simulink model "Filter_attivo"  (R2016b)
settings: Solver=ode23t  StartTime=0.0  StopTime=2.4  MaxStep=1e-4  RelTol=1e-3  EnableMultiTasking=on
values from neighbouring files (symbols this model uses):
  ampiezza_rete = 150/sqrt(3)    [Data.m]    (also in taratura.m)
  C = 2.2e-3    (= 0.0022)    [Data.m]
  C_raddr = 600e-6    (= 0.0006)    [Data.m]
  f = 50    [Data.m]    (also in Spettro_complesso.m = bar(-fp((26:25:25000-25)),PyTHD(length(PyTHD)-1:-1:length(Py)
  f_am = 500    [Data.m]
  h = Lagrange_coef(f,1/Tc)    [Data.m]    (also in Lagrange_coef.m = NaN(4,round(fc/f1*0.5)))
  h_rit = Lagrange_coef_rit(1.5)    [Data.m]
  k_interno = 0.99    [tuning.m]
  k_par_AM = 10    [Data.m]
  ki_PI = 0.2    [Data.m]
  ki_PLL = 1000    [Data.m]
  ki_ris = 47.5*2    (= 95)    [Data.m]
  kp_PI = 1.57    [Data.m]
  kp_PLL = 0.9    [Data.m]
  kp_ris = 47.5*0.089*2    (= 8.455)    [Data.m]
  L_disaccoppiamento = 2*1.18e-3    (= 0.00236)    [Data.m]    (also in taratura.m)
  L_rete = 4e-3    (= 0.004)    [Data.m]    (also in tuning.m)
  max_PI = 8    [Data.m]
  max_PLL = 1000    [Data.m]
  min_PI = -8    [Data.m]
  min_PLL = -1000    [Data.m]
  Notch_z = 1-Peaking_z    [Data.m]
  Notch_z_AM1 = 1-Peaking_z_AM1    [Notch.m]
  peak_rete = Peaking(f,1/Tc,0.1)    [Data.m]
  Peaking_dir1_d = c2d(Peaking_dir1_s,1/fs,'tustin')    [semipeaking.m]
  pendenza = 1000    [Data.m]
  R_carico = 50    [Data.m]
  R_disaccoppiamento = 2*13e-3    (= 0.026)    [Data.m]    (also in taratura.m)
  R_raddr = 60    [Data.m]
  R_rete = 100e-3    (= 0.1)    [Data.m]    (also in tuning.m = 0.01)
  T = 20e-3    (= 0.02)    [Data.m]    (also in tuning.m)
  tau_filtro_Vdc_ref = 0.15    [Data.m]
  Tc = 1/10000    (= 0.0001)    [Data.m]    (also in taratura.m; tuning.m)
  Vdc_ref = 200    [Data.m]    (also in taratura.m)
  w_filtro = 2*pi*f_taglio    (= 56548.6677646)    [Data.m]
undefined symbols (not defined in the file or in its folder): DiscIntNeverNeededParam, k_par, k_ser, Notch_z_AM1_5, Notch_z_AM1_7, Notch_z_AM2_5, Notch_z_AM2_7, Peaking_inv_d, plecs, Q_inv
libraries: powerlib x54, simulink x8, powerlib_extras x4, powerlib_meascontrol x2
(part 4 of 5)

== system Filter_attivo/Controllo tensione/Controllo ripetitivo/Controllo ripetitivo/Regolatore ripetitivo/Ripetitivo Modulazione AM/Scope2 ==
  1 : Inport
  " InputMux " : Subsystem
      mask Display: disp('Mux')
  " S-Function " : S-Function  FunctionName=plecs  SFunctionDeploymentMode=off  EnableBusSupport=off
  wires:
  1/1 -> " InputMux "/1(In1)
  " InputMux "/1(Out) -> " S-Function "/1

== system Filter_attivo/Controllo tensione/Controllo ripetitivo/Controllo ripetitivo/Regolatore ripetitivo/Ripetitivo Modulazione AM/notch_f_am ==
  In2 : Inport
  Enable : EnablePort  StatesWhenEnabling=reset
  Demux1 : Demux  Outputs=2
  Mux1 : Mux  Inputs=2
  notch_demodulazione_5_1 : Subsystem
  notch_demodulazione_5_7 : Subsystem
  Out1 : Outport
  wires:
  Demux1/2 -> notch_demodulazione_5_1/1(In1)
  In2/1 -> Demux1/1
  notch_demodulazione_5_1/1(Out1) -> Mux1/2
  notch_demodulazione_5_7/1(Out1) -> Mux1/1
  Demux1/1 -> notch_demodulazione_5_7/1(In1)
  Mux1/1 -> Out1/1

== system Filter_attivo/Controllo tensione/Controllo ripetitivo/Controllo ripetitivo/Regolatore ripetitivo/Scope/ InputMux  ==
  In1 : Inport
  Convert1 : DataTypeConversion  SaturateOnIntegerOverflow=on  RndMeth=Zero
  Mux : Mux  Inputs=1
  Out : Outport
  wires:
  Convert1/1 -> Mux/1
  In1/1 -> Convert1/1
  Mux/1 -> Out/1

== system Filter_attivo/Controllo tensione/Controllo ripetitivo/Controllo ripetitivo/Regolatore ripetitivo/vecchi controlli/ Ripetitivo buffer intero ==
  ir : Inport
  Add : Sum
  Add1 : Sum  Inputs=|-+
  Add2 : Sum  Inputs=|-+
  Delay1 : Delay  DelayLength=rit
  Delay2 : Delay  DelayLength=round((1/ro/f/Tc)-rit)
  Demux : Demux  Outputs=2
  Gain : Gain  Gain=-k_parallelo
  Gain1 : Gain  Gain=k_interno
  Gain3 : Gain  Gain=k_serie
  Mux : Mux  Inputs=2
  Scope : Subsystem  LoadFcn=plecs('sl', 300);  InitFcn=plecs('sl', 314);  StartFcn=plecs('sl', 308);  StopFcn=plecs('sl', 309);  mask{Settings=<binary blob, 424 chars, not shown>}
      mask init:
      | plecs('sl', 315);
      settings: CopyFcn=plecs('sl', 303);  DeleteFcn=plecs('sl', 305);  UndoDeleteFcn=plecs('sl', 306);  PreSaveFcn=plecs('sl', 311);  NameChangeFcn=plecs('sl', 310);  DestroyFcn=plecs('sl', 307);  OpenFcn=plecs('sl', 302);  ErrorFcn=plerrorfcn
      mask Display: plot([0.1 0.9 0.9 0.1 0.1], [0.9 0.9 0.5 0.5 0.9])
  Sum : Sum  Inputs=|-+
  ir* : Constant  Value=0
  k_serie step : Subsystem  mask{k_serie_partenza=0.8, passo_t=0.5, passo_y=0.01}
      mask prompts: k_serie_partenza "partenza della costante"; passo_t "step dei tempi"; passo_y "step di costante"
  Out : Outport
  wires:
  Add/1 -> Scope/3(3), Out/1
  Gain/1 -> Add/1
  ir/1 -> Demux/1
  Demux/2 -> Add1/1
  Demux/1 -> Add2/1
  ir*/1 -> Add2/2, Add1/2
  Add2/1 -> Mux/1
  Add1/1 -> Mux/2
  Mux/1 -> Gain/1, Sum/1, Scope/1(1)
  Delay1/1 -> Gain1/1
  Delay2/1 -> Gain3/1, Delay1/1
  Sum/1 -> Delay2/1
  Gain1/1 -> Sum/2
  Gain3/1 -> Add/2

== system Filter_attivo/Controllo tensione/Controllo ripetitivo/Controllo ripetitivo/Regolatore ripetitivo/vecchi controlli/ Ripetitivo buffer intero1.5 di ritardo ==
  ir : Inport
  Add : Sum
  Add1 : Sum  Inputs=|-+
  Add2 : Sum  Inputs=|-+
  Delay1 : Delay  DelayLength=rit
  Delay2 : Delay  DelayLength=round((1/ro/f/Tc)-3-rit)
  Demux : Demux  Outputs=2
  Gain : Gain  Gain=-k_parallelo
  Gain1 : Gain  Gain=k_interno
  Gain2 : Gain  Gain=k_serie
  Mux : Mux  Inputs=2
  Scope : Subsystem  LoadFcn=plecs('sl', 300);  InitFcn=plecs('sl', 314);  StartFcn=plecs('sl', 308);  StopFcn=plecs('sl', 309);  mask{Settings=<binary blob, 424 chars, not shown>}
      mask init:
      | plecs('sl', 315);
      settings: CopyFcn=plecs('sl', 303);  DeleteFcn=plecs('sl', 305);  UndoDeleteFcn=plecs('sl', 306);  PreSaveFcn=plecs('sl', 311);  NameChangeFcn=plecs('sl', 310);  DestroyFcn=plecs('sl', 307);  OpenFcn=plecs('sl', 302);  ErrorFcn=plerrorfcn
      mask Display: plot([0.1 0.9 0.9 0.1 0.1], [0.9 0.9 0.5 0.5 0.9])
  Sum : Sum  Inputs=|-+
  ir* : Constant  Value=0
  k_serie step : Subsystem  mask{k_serie_partenza=5, passo_t=0.6, passo_y=0}
      mask prompts: k_serie_partenza "partenza della costante"; passo_t "step dei tempi"; passo_y "step di costante"
  ritardo 1.5 : DiscreteFir  Coefficients=[h_rit(1) h_rit(2) h_rit(3) h_rit(4)]
  ritardo di 1.5 : DiscreteFir  Coefficients=[h_rit(1) h_rit(2) h_rit(3) h_rit(4)]
  Out : Outport
  wires:
  Gain1/1 -> Sum/2
  Sum/1 -> Delay2/1
  Delay2/1 -> ritardo di 1.5/1
  ritardo 1.5/1 -> Gain1/1
  Mux/1 -> Gain/1, Scope/1(1), Sum/1
  Add1/1 -> Mux/2
  Add2/1 -> Mux/1
  ir*/1 -> Add1/2, Add2/2
  Demux/1 -> Add2/1
  Demux/2 -> Add1/1
  ir/1 -> Demux/1
  Gain/1 -> Add/1
  Add/1 -> Out/1, Scope/3(3)
  ritardo di 1.5/1 -> Gain2/1, Delay1/1
  Gain2/1 -> Scope/2(2), Add/2
  Delay1/1 -> ritardo 1.5/1

== system Filter_attivo/Controllo tensione/Controllo ripetitivo/Controllo ripetitivo/Regolatore ripetitivo/vecchi controlli/ Ripetitivo stazionario ==
  ir : Inport
  Add : Sum
  Add1 : Sum  Inputs=|-+
  Add2 : Sum  Inputs=|-+
  Delay1 : Delay  DelayLength=rit
  Delay2 : Delay  DelayLength=round((1/ro/f/Tc)-rit)
  Demux : Demux  Outputs=2
  Gain : Gain  Gain=-k_par
  Gain1 : Gain  Gain=k_interno
  Gain2 : Gain  Gain=k_ser
  Mux : Mux  Inputs=2
  Scope : Subsystem  LoadFcn=plecs('sl', 300);  InitFcn=plecs('sl', 314);  StartFcn=plecs('sl', 308);  StopFcn=plecs('sl', 309);  mask{Settings=<binary blob, 424 chars, not shown>}
      mask init:
      | plecs('sl', 315);
      settings: CopyFcn=plecs('sl', 303);  DeleteFcn=plecs('sl', 305);  UndoDeleteFcn=plecs('sl', 306);  PreSaveFcn=plecs('sl', 311);  NameChangeFcn=plecs('sl', 310);  DestroyFcn=plecs('sl', 307);  OpenFcn=plecs('sl', 302);  ErrorFcn=plerrorfcn
      mask Display: plot([0.1 0.9 0.9 0.1 0.1], [0.9 0.9 0.5 0.5 0.9])
  Sum : Sum  Inputs=|+-
  ir* : Constant  Value=0
  Out : Outport
  wires:
  Gain1/1 -> Sum/2
  Sum/1 -> Delay2/1
  Delay2/1 -> Delay1/1, Gain2/1
  Delay1/1 -> Gain1/1
  Mux/1 -> Scope/1(1), Sum/1, Gain/1
  Add1/1 -> Mux/2
  Add2/1 -> Mux/1
  ir*/1 -> Add1/2, Add2/2
  Demux/1 -> Add2/1
  Demux/2 -> Add1/1
  ir/1 -> Demux/1
  Gain/1 -> Add/1
  Add/1 -> Out/1, Scope/3(3)
  Gain2/1 -> Add/2, Scope/2(2)

== system Filter_attivo/Controllo tensione/Controllo ripetitivo/Controllo ripetitivo/Regolatore ripetitivo/vecchi controlli/ buffer intero mattavelli buchi amplificati ==
  e : Inport
  Add : Sum
  Delay2 : Delay  DelayLength=round((1/ro/f/Tc)-1)
  Delay3 : Delay  DelayLength=round((1/ro/f/Tc)-rit)
  Discrete Transfer Fcn : DiscreteTransferFcn  Numerator=cell2mat(Q_inv.num)  Denominator=cell2mat(Q_inv.den)
  Gain2 : Gain  Gain=k_serie
  Q : DiscreteFir  Coefficients=[0.05 0.9 0.05]
  Scope : Subsystem  LoadFcn=plecs('sl', 300);  InitFcn=plecs('sl', 314);  StartFcn=plecs('sl', 308);  StopFcn=plecs('sl', 309);  mask{Settings=<binary blob, 216 chars, not shown>}
      mask init:
      | plecs('sl', 315);
      settings: CopyFcn=plecs('sl', 303);  DeleteFcn=plecs('sl', 305);  UndoDeleteFcn=plecs('sl', 306);  PreSaveFcn=plecs('sl', 311);  NameChangeFcn=plecs('sl', 310);  DestroyFcn=plecs('sl', 307);  OpenFcn=plecs('sl', 302);  ErrorFcn=plerrorfcn
      mask Display: plot([0.1 0.9 0.9 0.1 0.1], [0.9 0.9 0.5 0.5 0.9])
  Sum : Sum  Inputs=|++
  Sum1 : Sum  Inputs=|++
  Sum2 : Sum
  k_serie step : Subsystem  mask{k_serie_partenza=5, passo_t=0.6, passo_y=0}
      mask prompts: k_serie_partenza "partenza della costante"; passo_t "step dei tempi"; passo_y "step di costante"
  Out : Outport
  wires:
  Sum2/1 -> Out/1
  Gain2/1 -> Sum2/2
  e/1 -> Scope/1(1), Sum/1, Sum2/1
  Sum/1 -> Delay2/1
  Delay2/1 -> Q/1
  Q/1 -> Delay3/1, Sum1/2, Sum/2
  Delay3/1 -> Sum1/1
  Sum1/1 -> Discrete Transfer Fcn/1
  Discrete Transfer Fcn/1 -> Gain2/1

== system Filter_attivo/Controllo tensione/Controllo ripetitivo/Controllo ripetitivo/Regolatore ripetitivo/vecchi controlli/Generatore step  ==
  In1 : Inport
  Constant : Constant  Value=Tc
  Constant1 : Constant  Value=k_serie_partenza
  Constant2 : Constant  Value=passo_t
  Constant3 : Constant  Value=passo_y
  MATLAB Function : MATLAB Function  TreatAsAtomicUnit=on
  Product : Product
  Out1 : Outport
  wires:
  Constant/1 -> MATLAB Function/1(Tc)
  Constant2/1 -> MATLAB Function/3(step_t)
  Constant1/1 -> MATLAB Function/2(k_partenza)
  Constant3/1 -> MATLAB Function/4(step_y)
  In1/1 -> Product/1
  MATLAB Function/1(y) -> Product/2
  Product/1 -> Out1/1

== system Filter_attivo/Controllo tensione/Controllo ripetitivo/Controllo ripetitivo/Regolatore ripetitivo/vecchi controlli/Ripetitivo Modulazione AM1 ==
  In1 : Inport
  Add : Sum
  Add1 : Sum  Inputs=|-+
  Add2 : Sum  Inputs=|-+
  Banco di ripetitivi : Subsystem
  Banco notch 5_7_AM : Subsystem
  Constant : Constant  Value=f_am
  Demux : Demux  Outputs=2
  Divide : Product  Inputs=**
  Divide1 : Product  Inputs=**
  Gain : Gain  Gain=-k_par_AM
  Gain3 : Gain  Gain=2*pi
  Integratore discreto con reset a 2*pi : Subsystem
  Mux : Mux  Inputs=2
  Scope : Subsystem  LoadFcn=plecs('sl', 300);  InitFcn=plecs('sl', 314);  StartFcn=plecs('sl', 308);  StopFcn=plecs('sl', 309);  mask{Settings=<binary blob, 424 chars, not shown>}
      mask init:
      | plecs('sl', 315);
      settings: CopyFcn=plecs('sl', 303);  DeleteFcn=plecs('sl', 305);  UndoDeleteFcn=plecs('sl', 306);  PreSaveFcn=plecs('sl', 311);  NameChangeFcn=plecs('sl', 310);  DestroyFcn=plecs('sl', 307);  OpenFcn=plecs('sl', 302);  ErrorFcn=plerrorfcn
      mask Display: plot([0.1 0.9 0.9 0.1 0.1], [0.9 0.9 0.5 0.5 0.9])
  Scope1 : Subsystem  LoadFcn=plecs('sl', 300);  InitFcn=plecs('sl', 314);  StartFcn=plecs('sl', 308);  StopFcn=plecs('sl', 309);  mask{Settings=<binary blob, 216 chars, not shown>}
      mask init:
      | plecs('sl', 315);
      settings: CopyFcn=plecs('sl', 303);  DeleteFcn=plecs('sl', 305);  UndoDeleteFcn=plecs('sl', 306);  PreSaveFcn=plecs('sl', 311);  NameChangeFcn=plecs('sl', 310);  DestroyFcn=plecs('sl', 307);  OpenFcn=plecs('sl', 302);  ErrorFcn=plerrorfcn
      mask Display: plot([0.1 0.9 0.9 0.1 0.1], [0.9 0.9 0.5 0.5 0.9])
  Trigonometric Function : Trigonometry  Operator=cos
  ir* : Constant  Value=0
  Out1 : Outport
  wires:
  Integratore discreto con reset a 2*pi/1(teta) -> Trigonometric Function/1
  Banco notch 5_7_AM/1(Out1) -> Add/2, Scope/2(2)
  Divide1/1 -> Banco notch 5_7_AM/1(In2)
  Mux/1 -> Divide/1, Gain/1, Scope/1(1)
  Demux/2 -> Add1/1
  Add2/1 -> Mux/1
  In1/1 -> Demux/1
  Demux/1 -> Add2/1
  Add/1 -> Scope/3(3), Out1/1
  ir*/1 -> Add1/2, Add2/2
  Add1/1 -> Mux/2
  Gain3/1 -> Integratore discreto con reset a 2*pi/1(omega)
  Trigonometric Function/1 -> Scope1/1(1), Divide1/2, Divide/2
  Banco di ripetitivi/1(Out1) -> Divide1/1
  Constant/1 -> Gain3/1
  Divide/1 -> Banco di ripetitivi/1(In1)
  Gain/1 -> Add/1

== system Filter_attivo/Controllo tensione/Controllo ripetitivo/Controllo ripetitivo con downsampling/Regolatore ripetitivo/ buffer intero fase zero/Scope ==
  1 : Inport
  2 : Inport  Port=2
  3 : Inport  Port=3
  " 1 " : DataTypeConversion  SaturateOnIntegerOverflow=on  RndMeth=Zero
  " 2 " : DataTypeConversion  SaturateOnIntegerOverflow=on  RndMeth=Zero
  " 3 " : DataTypeConversion  SaturateOnIntegerOverflow=on  RndMeth=Zero
  " InputMux " : Mux  Inputs=3
  " S-Function " : S-Function  FunctionName=plecs  SFunctionDeploymentMode=off  EnableBusSupport=off
  wires:
  " InputMux "/1 -> " S-Function "/1
  1/1 -> " 1 "/1
  " 1 "/1 -> " InputMux "/1
  2/1 -> " 2 "/1
  " 2 "/1 -> " InputMux "/2
  3/1 -> " 3 "/1
  " 3 "/1 -> " InputMux "/3

== system Filter_attivo/Controllo tensione/Controllo ripetitivo/Controllo ripetitivo con downsampling/Regolatore ripetitivo/ buffer metà fase zero/Scope ==
  1 : Inport
  2 : Inport  Port=2
  3 : Inport  Port=3
  " 1 " : DataTypeConversion  SaturateOnIntegerOverflow=on  RndMeth=Zero
  " 2 " : DataTypeConversion  SaturateOnIntegerOverflow=on  RndMeth=Zero
  " 3 " : DataTypeConversion  SaturateOnIntegerOverflow=on  RndMeth=Zero
  " InputMux " : Mux  Inputs=3
  " S-Function " : S-Function  FunctionName=plecs  SFunctionDeploymentMode=off  EnableBusSupport=off
  wires:
  " InputMux "/1 -> " S-Function "/1
  1/1 -> " 1 "/1
  " 1 "/1 -> " InputMux "/1
  2/1 -> " 2 "/1
  " 2 "/1 -> " InputMux "/2
  3/1 -> " 3 "/1
  " 3 "/1 -> " InputMux "/3

== system Filter_attivo/Controllo tensione/Controllo ripetitivo/Controllo ripetitivo con downsampling/Regolatore ripetitivo/ buffer metà fase zero/k_serie step ==
  In1 : Inport
  Constant : Constant  Value=Tc
  Constant1 : Constant  Value=k_serie_partenza
  Constant2 : Constant  Value=passo_t
  Constant3 : Constant  Value=passo_y
  MATLAB Function : MATLAB Function  TreatAsAtomicUnit=on
  Product : Product
  Out1 : Outport
  wires:
  Constant/1 -> MATLAB Function/1(Tc)
  Constant2/1 -> MATLAB Function/3(step_t)
  Constant1/1 -> MATLAB Function/2(k_partenza)
  Constant3/1 -> MATLAB Function/4(step_y)
  In1/1 -> Product/1
  MATLAB Function/1(k) -> Product/2
  Product/1 -> Out1/1

== system Filter_attivo/Controllo tensione/Controllo ripetitivo/Controllo ripetitivo con downsampling/Regolatore ripetitivo/ buffer metà fase zero-riduzione di 3/Scope ==
  1 : Inport
  2 : Inport  Port=2
  3 : Inport  Port=3
  " 1 " : DataTypeConversion  SaturateOnIntegerOverflow=on  RndMeth=Zero
  " 2 " : DataTypeConversion  SaturateOnIntegerOverflow=on  RndMeth=Zero
  " 3 " : DataTypeConversion  SaturateOnIntegerOverflow=on  RndMeth=Zero
  " InputMux " : Mux  Inputs=3
  " S-Function " : S-Function  FunctionName=plecs  SFunctionDeploymentMode=off  EnableBusSupport=off
  wires:
  " 3 "/1 -> " InputMux "/3
  3/1 -> " 3 "/1
  " 2 "/1 -> " InputMux "/2
  2/1 -> " 2 "/1
  " 1 "/1 -> " InputMux "/1
  1/1 -> " 1 "/1
  " InputMux "/1 -> " S-Function "/1

== system Filter_attivo/Controllo tensione/Controllo ripetitivo/Controllo ripetitivo con downsampling/Regolatore ripetitivo/ buffer metà fase zero-riduzione di 3/k_serie step ==
  In1 : Inport
  Constant : Constant  Value=Tc
  Constant1 : Constant  Value=k_serie_partenza
  Constant2 : Constant  Value=passo_t
  Constant3 : Constant  Value=passo_y
  MATLAB Function : MATLAB Function  TreatAsAtomicUnit=on
  Product : Product
  Out1 : Outport
  wires:
  Product/1 -> Out1/1
  MATLAB Function/1(k) -> Product/2
  In1/1 -> Product/1
  Constant3/1 -> MATLAB Function/4(step_y)
  Constant1/1 -> MATLAB Function/2(k_partenza)
  Constant2/1 -> MATLAB Function/3(step_t)
  Constant/1 -> MATLAB Function/1(Tc)

== system Filter_attivo/Controllo tensione/Controllo ripetitivo/Controllo ripetitivo con downsampling/Regolatore ripetitivo/ buffer metà mattavelli/Scope ==
  1 : Inport
  " InputMux " : Subsystem
      mask Display: disp('Mux')
  " S-Function " : S-Function  FunctionName=plecs  SFunctionDeploymentMode=off  EnableBusSupport=off
  wires:
  " InputMux "/1(Out) -> " S-Function "/1
  1/1 -> " InputMux "/1(In1)

== system Filter_attivo/Controllo tensione/Controllo ripetitivo/Controllo ripetitivo con downsampling/Regolatore ripetitivo/ buffer metà mattavelli/k_serie step ==
  In1 : Inport
  Constant : Constant  Value=Tc
  Constant1 : Constant  Value=k_serie_partenza
  Constant2 : Constant  Value=passo_t
  Constant3 : Constant  Value=passo_y
  MATLAB Function : MATLAB Function  TreatAsAtomicUnit=on
  Product : Product
  Out1 : Outport
  wires:
  Constant/1 -> MATLAB Function/1(Tc)
  Constant2/1 -> MATLAB Function/3(step_t)
  Constant1/1 -> MATLAB Function/2(k_partenza)
  Constant3/1 -> MATLAB Function/4(step_y)
  In1/1 -> Product/1
  MATLAB Function/1(k) -> Product/2
  Product/1 -> Out1/1

== system Filter_attivo/Controllo tensione/Controllo ripetitivo/Controllo ripetitivo con downsampling/Regolatore ripetitivo/Scope/ InputMux  ==
  In1 : Inport
  Convert1 : DataTypeConversion  SaturateOnIntegerOverflow=on  RndMeth=Zero
  Mux : Mux  Inputs=1
  Out : Outport
  wires:
  Convert1/1 -> Mux/1
  In1/1 -> Convert1/1
  Mux/1 -> Out/1

== system Filter_attivo/Controllo tensione/Controllo PR 10 kHz/PLL_tempo_discreto/Subsystem/FILTRO peaking diretta_prima/Scope/ InputMux  ==
  In1 : Inport
  Convert1 : DataTypeConversion  SaturateOnIntegerOverflow=on  RndMeth=Zero
  Mux : Mux  Inputs=1
  Out : Outport
  wires:
  Convert1/1 -> Mux/1
  In1/1 -> Convert1/1
  Mux/1 -> Out/1

== system Filter_attivo/Controllo tensione/Controllo PR 10 kHz/PLL_tempo_discreto/Subsystem/notch_prima_tensione/FILTRO peaking diretta_prima/Scope ==
  1 : Inport
  " InputMux " : Subsystem
      mask Display: disp('Mux')
  " S-Function " : S-Function  FunctionName=plecs  SFunctionDeploymentMode=off  EnableBusSupport=off
  wires:
  1/1 -> " InputMux "/1(In1)
  " InputMux "/1(Out) -> " S-Function "/1

== system Filter_attivo/Controllo tensione/Controllo ripetitivo/Controllo ripetitivo/Regolatore ripetitivo/ buffer intero feedforward/Scope/ InputMux  ==
  In1 : Inport
  Convert1 : DataTypeConversion  SaturateOnIntegerOverflow=on  RndMeth=Zero
  Mux : Mux  Inputs=1
  Out : Outport
  wires:
  Convert1/1 -> Mux/1
  In1/1 -> Convert1/1
  Mux/1 -> Out/1

== system Filter_attivo/Controllo tensione/Controllo ripetitivo/Controllo ripetitivo/Regolatore ripetitivo/ buffer intero feedforward/Scope1/ InputMux  ==
  In1 : Inport
  Convert1 : DataTypeConversion  SaturateOnIntegerOverflow=on  RndMeth=Zero
  Mux : Mux  Inputs=1
  Out : Outport
  wires:
  Mux/1 -> Out/1
  In1/1 -> Convert1/1
  Convert1/1 -> Mux/1

== system Filter_attivo/Controllo tensione/Controllo ripetitivo/Controllo ripetitivo/Regolatore ripetitivo/ buffer metà feedforward/Scope/ InputMux  ==
  In1 : Inport
  Convert1 : DataTypeConversion  SaturateOnIntegerOverflow=on  RndMeth=Zero
  Mux : Mux  Inputs=1
  Out : Outport
  wires:
  Mux/1 -> Out/1
  In1/1 -> Convert1/1
  Convert1/1 -> Mux/1

== system Filter_attivo/Controllo tensione/Controllo ripetitivo/Controllo ripetitivo/Regolatore ripetitivo/Ripetitivo Modulazione AM/Banco di ripetitivi/Subsystem ==
  In1 : Inport
  In2 : Inport  Port=2
  In3 : Inport  Port=3
  In4 : Inport  Port=4
  In5 : Inport  Port=5
  In6 : Inport  Port=6
  Gain : Gain  Gain=abilitatore5
  Gain1 : Gain  Gain=abilitatore7
  Gain2 : Gain  Gain=abilitatore13
  Gain3 : Gain  Gain=abilitatore11
  Gain4 : Gain  Gain=abilitatore17
  Gain5 : Gain  Gain=abilitatore19
  Sum : Sum  Inputs=++++++
  Out1 : Outport
  wires:
  In5/1 -> Gain4/1
  In3/1 -> Gain3/1
  In1/1 -> Gain/1
  In2/1 -> Gain1/1
  In4/1 -> Gain2/1
  In6/1 -> Gain5/1
  Sum/1 -> Out1/1
  Gain/1 -> Sum/1
  Gain1/1 -> Sum/2
  Gain3/1 -> Sum/3
  Gain2/1 -> Sum/4
  Gain4/1 -> Sum/5
  Gain5/1 -> Sum/6

== system Filter_attivo/Controllo tensione/Controllo ripetitivo/Controllo ripetitivo/Regolatore ripetitivo/Ripetitivo Modulazione AM/Banco di ripetitivi/rep_comp 1 ==
  In1 : Inport
  Add1 : Sum  Inputs=-+
  Delay1 : Delay
  Delay3 : Delay  DelayLength=fix(1/(Tc*f*1*ro)-1-rit)
  Discrete FIR Filter : DiscreteFir  Coefficients=[h(1,ro) h(2,ro) h(3,ro) h(4,ro)]
  Gain : Gain  Gain=0.98
  Gain1 : Gain  Gain=g_interno
  Scope2 : Subsystem  LoadFcn=plecs('sl', 300);  InitFcn=plecs('sl', 314);  StartFcn=plecs('sl', 308);  StopFcn=plecs('sl', 309);  mask{Settings=<binary blob, 216 chars, not shown>}
      mask init:
      | plecs('sl', 315);
      settings: CopyFcn=plecs('sl', 303);  DeleteFcn=plecs('sl', 305);  UndoDeleteFcn=plecs('sl', 306);  PreSaveFcn=plecs('sl', 311);  NameChangeFcn=plecs('sl', 310);  DestroyFcn=plecs('sl', 307);  OpenFcn=plecs('sl', 302);  ErrorFcn=plerrorfcn
      mask Display: plot([0.1 0.9 0.9 0.1 0.1], [0.9 0.9 0.5 0.5 0.9])
  Out1 : Outport
  wires:
  Delay3/1 -> Discrete FIR Filter/1
  In1/1 -> Add1/1
  Add1/1 -> Delay3/1
  Delay1/1 -> Add1/2
  Gain/1 -> Delay1/1
  Discrete FIR Filter/1 -> Gain1/1, Gain/1
  Gain1/1 -> Scope2/1(1), Out1/1

== system Filter_attivo/Controllo tensione/Controllo ripetitivo/Controllo ripetitivo/Regolatore ripetitivo/Ripetitivo Modulazione AM/Banco di ripetitivi/rep_comp 2 ==
  In1 : Inport
  Add1 : Sum  Inputs=-+
  Delay1 : Delay
  Delay3 : Delay  DelayLength=fix(1/(Tc*f*1*ro)-1-rit)
  Discrete FIR Filter : DiscreteFir  Coefficients=[h(1,ro) h(2,ro) h(3,ro) h(4,ro)]
  Gain : Gain  Gain=0.98
  Gain1 : Gain  Gain=g_interno
  Scope2 : Subsystem  LoadFcn=plecs('sl', 300);  InitFcn=plecs('sl', 314);  StartFcn=plecs('sl', 308);  StopFcn=plecs('sl', 309);  mask{Settings=<binary blob, 216 chars, not shown>}
      mask init:
      | plecs('sl', 315);
      settings: CopyFcn=plecs('sl', 303);  DeleteFcn=plecs('sl', 305);  UndoDeleteFcn=plecs('sl', 306);  PreSaveFcn=plecs('sl', 311);  NameChangeFcn=plecs('sl', 310);  DestroyFcn=plecs('sl', 307);  OpenFcn=plecs('sl', 302);  ErrorFcn=plerrorfcn
      mask Display: plot([0.1 0.9 0.9 0.1 0.1], [0.9 0.9 0.5 0.5 0.9])
  Out1 : Outport
  wires:
  Gain1/1 -> Out1/1, Scope2/1(1)
  Discrete FIR Filter/1 -> Gain/1, Gain1/1
  Gain/1 -> Delay1/1
  Delay1/1 -> Add1/2
  Add1/1 -> Delay3/1
  In1/1 -> Add1/1
  Delay3/1 -> Discrete FIR Filter/1

== system Filter_attivo/Controllo tensione/Controllo ripetitivo/Controllo ripetitivo/Regolatore ripetitivo/Ripetitivo Modulazione AM/Banco di ripetitivi/rep_comp 3 ==
  In1 : Inport
  Add1 : Sum  Inputs=-+
  Delay1 : Delay
  Delay3 : Delay  DelayLength=fix(1/(Tc*f*1*ro)-1-rit)
  Discrete FIR Filter : DiscreteFir  Coefficients=[h(1,ro) h(2,ro) h(3,ro) h(4,ro)]
  Gain : Gain  Gain=0.98
  Gain1 : Gain  Gain=g_interno
  Scope2 : Subsystem  LoadFcn=plecs('sl', 300);  InitFcn=plecs('sl', 314);  StartFcn=plecs('sl', 308);  StopFcn=plecs('sl', 309);  mask{Settings=<binary blob, 216 chars, not shown>}
      mask init:
      | plecs('sl', 315);
      settings: CopyFcn=plecs('sl', 303);  DeleteFcn=plecs('sl', 305);  UndoDeleteFcn=plecs('sl', 306);  PreSaveFcn=plecs('sl', 311);  NameChangeFcn=plecs('sl', 310);  DestroyFcn=plecs('sl', 307);  OpenFcn=plecs('sl', 302);  ErrorFcn=plerrorfcn
      mask Display: plot([0.1 0.9 0.9 0.1 0.1], [0.9 0.9 0.5 0.5 0.9])
  Out1 : Outport
  wires:
  Delay3/1 -> Discrete FIR Filter/1
  In1/1 -> Add1/1
  Add1/1 -> Delay3/1
  Delay1/1 -> Add1/2
  Gain/1 -> Delay1/1
  Discrete FIR Filter/1 -> Gain1/1, Gain/1
  Gain1/1 -> Scope2/1(1), Out1/1

== system Filter_attivo/Controllo tensione/Controllo ripetitivo/Controllo ripetitivo/Regolatore ripetitivo/Ripetitivo Modulazione AM/Banco di ripetitivi/rep_comp 4 ==
  In1 : Inport
  Add1 : Sum  Inputs=-+
  Delay1 : Delay
  Delay3 : Delay  DelayLength=fix(1/(Tc*f*1*ro)-1-rit)
  Discrete FIR Filter : DiscreteFir  Coefficients=[h(1,ro) h(2,ro) h(3,ro) h(4,ro)]
  Gain : Gain  Gain=0.98
  Gain1 : Gain  Gain=g_interno
  Scope2 : Subsystem  LoadFcn=plecs('sl', 300);  InitFcn=plecs('sl', 314);  StartFcn=plecs('sl', 308);  StopFcn=plecs('sl', 309);  mask{Settings=<binary blob, 216 chars, not shown>}
      mask init:
      | plecs('sl', 315);
      settings: CopyFcn=plecs('sl', 303);  DeleteFcn=plecs('sl', 305);  UndoDeleteFcn=plecs('sl', 306);  PreSaveFcn=plecs('sl', 311);  NameChangeFcn=plecs('sl', 310);  DestroyFcn=plecs('sl', 307);  OpenFcn=plecs('sl', 302);  ErrorFcn=plerrorfcn
      mask Display: plot([0.1 0.9 0.9 0.1 0.1], [0.9 0.9 0.5 0.5 0.9])
  Out1 : Outport
  wires:
  Gain1/1 -> Out1/1, Scope2/1(1)
  Discrete FIR Filter/1 -> Gain/1, Gain1/1
  Gain/1 -> Delay1/1
  Delay1/1 -> Add1/2
  Add1/1 -> Delay3/1
  In1/1 -> Add1/1
  Delay3/1 -> Discrete FIR Filter/1

== system Filter_attivo/Controllo tensione/Controllo ripetitivo/Controllo ripetitivo/Regolatore ripetitivo/Ripetitivo Modulazione AM/Banco di ripetitivi/rep_comp 5 ==
  In1 : Inport
  Add1 : Sum  Inputs=-+
  Delay1 : Delay
  Delay3 : Delay  DelayLength=fix(1/(Tc*f*1*ro)-1-rit)
  Discrete FIR Filter : DiscreteFir  Coefficients=[h(1,ro) h(2,ro) h(3,ro) h(4,ro)]
  Gain : Gain  Gain=0.98
  Gain1 : Gain  Gain=g_interno
  Scope2 : Subsystem  LoadFcn=plecs('sl', 300);  InitFcn=plecs('sl', 314);  StartFcn=plecs('sl', 308);  StopFcn=plecs('sl', 309);  mask{Settings=<binary blob, 216 chars, not shown>}
      mask init:
      | plecs('sl', 315);
      settings: CopyFcn=plecs('sl', 303);  DeleteFcn=plecs('sl', 305);  UndoDeleteFcn=plecs('sl', 306);  PreSaveFcn=plecs('sl', 311);  NameChangeFcn=plecs('sl', 310);  DestroyFcn=plecs('sl', 307);  OpenFcn=plecs('sl', 302);  ErrorFcn=plerrorfcn
      mask Display: plot([0.1 0.9 0.9 0.1 0.1], [0.9 0.9 0.5 0.5 0.9])
  Out1 : Outport
  wires:
  Delay3/1 -> Discrete FIR Filter/1
  In1/1 -> Add1/1
  Add1/1 -> Delay3/1
  Delay1/1 -> Add1/2
  Gain/1 -> Delay1/1
  Discrete FIR Filter/1 -> Gain1/1, Gain/1
  Gain1/1 -> Scope2/1(1), Out1/1

== system Filter_attivo/Controllo tensione/Controllo ripetitivo/Controllo ripetitivo/Regolatore ripetitivo/Ripetitivo Modulazione AM/Banco di ripetitivi/rep_comp 6 ==
  In1 : Inport
  Add1 : Sum  Inputs=-+
  Delay1 : Delay
  Delay3 : Delay  DelayLength=fix(1/(Tc*f*1*ro)-1-rit)
  Discrete FIR Filter : DiscreteFir  Coefficients=[h(1,ro) h(2,ro) h(3,ro) h(4,ro)]
  Gain : Gain  Gain=0.98
  Gain1 : Gain  Gain=g_interno
  Scope2 : Subsystem  LoadFcn=plecs('sl', 300);  InitFcn=plecs('sl', 314);  StartFcn=plecs('sl', 308);  StopFcn=plecs('sl', 309);  mask{Settings=<binary blob, 216 chars, not shown>}
      mask init:
      | plecs('sl', 315);
      settings: CopyFcn=plecs('sl', 303);  DeleteFcn=plecs('sl', 305);  UndoDeleteFcn=plecs('sl', 306);  PreSaveFcn=plecs('sl', 311);  NameChangeFcn=plecs('sl', 310);  DestroyFcn=plecs('sl', 307);  OpenFcn=plecs('sl', 302);  ErrorFcn=plerrorfcn
      mask Display: plot([0.1 0.9 0.9 0.1 0.1], [0.9 0.9 0.5 0.5 0.9])
  Out1 : Outport
  wires:
  Gain1/1 -> Out1/1, Scope2/1(1)
  Discrete FIR Filter/1 -> Gain/1, Gain1/1
  Gain/1 -> Delay1/1
  Delay1/1 -> Add1/2
  Add1/1 -> Delay3/1
  In1/1 -> Add1/1
  Delay3/1 -> Discrete FIR Filter/1

== system Filter_attivo/Controllo tensione/Controllo ripetitivo/Controllo ripetitivo/Regolatore ripetitivo/Ripetitivo Modulazione AM/Banco notch 5_7_AM/notch_demodulazione_5_1 ==
  In1 : Inport
  Discrete Transfer Fcn : DiscreteTransferFcn  Numerator=cell2mat(Notch_z_AM1_5.num)  Denominator=cell2mat(Notch_z_AM1_5.den)
  Discrete Transfer Fcn1 : DiscreteTransferFcn  Numerator=cell2mat(Notch_z_AM1.num)  Denominator=cell2mat(Notch_z_AM1.den)
  Discrete Transfer Fcn2 : DiscreteTransferFcn  Numerator=cell2mat(Notch_z_AM1_7.num)  Denominator=cell2mat(Notch_z_AM1_7.den)
  Out1 : Outport
  wires:
  Discrete Transfer Fcn1/1 -> Out1/1
  Discrete Transfer Fcn2/1 -> Discrete Transfer Fcn1/1
  Discrete Transfer Fcn/1 -> Discrete Transfer Fcn2/1
  In1/1 -> Discrete Transfer Fcn/1

== system Filter_attivo/Controllo tensione/Controllo ripetitivo/Controllo ripetitivo/Regolatore ripetitivo/Ripetitivo Modulazione AM/Banco notch 5_7_AM/notch_demodulazione_5_7 ==
  In1 : Inport
  Discrete Transfer Fcn : DiscreteTransferFcn  Numerator=cell2mat(Notch_z_AM1_5.num)  Denominator=cell2mat(Notch_z_AM1_5.den)
  Discrete Transfer Fcn1 : DiscreteTransferFcn  Numerator=cell2mat(Notch_z_AM1.num)  Denominator=cell2mat(Notch_z_AM1.den)
  Discrete Transfer Fcn2 : DiscreteTransferFcn  Numerator=cell2mat(Notch_z_AM1_7.num)  Denominator=cell2mat(Notch_z_AM1_7.den)
  Out1 : Outport
  wires:
  In1/1 -> Discrete Transfer Fcn/1
  Discrete Transfer Fcn/1 -> Discrete Transfer Fcn2/1
  Discrete Transfer Fcn2/1 -> Discrete Transfer Fcn1/1
  Discrete Transfer Fcn1/1 -> Out1/1

== system Filter_attivo/Controllo tensione/Controllo ripetitivo/Controllo ripetitivo/Regolatore ripetitivo/Ripetitivo Modulazione AM/Scope2/ InputMux  ==
  In1 : Inport
  Convert1 : DataTypeConversion  SaturateOnIntegerOverflow=on  RndMeth=Zero
  Mux : Mux  Inputs=1
  Out : Outport
  wires:
  Convert1/1 -> Mux/1
  In1/1 -> Convert1/1
  Mux/1 -> Out/1

== system Filter_attivo/Controllo tensione/Controllo ripetitivo/Controllo ripetitivo/Regolatore ripetitivo/Ripetitivo Modulazione AM/notch_f_am/notch_demodulazione_5_1 ==
  In1 : Inport
  Discrete Transfer Fcn1 : DiscreteTransferFcn  Numerator=cell2mat(Notch_z_AM1.num)  Denominator=cell2mat(Notch_z_AM1.den)
  Out1 : Outport
  wires:
  In1/1 -> Discrete Transfer Fcn1/1
  Discrete Transfer Fcn1/1 -> Out1/1

== system Filter_attivo/Controllo tensione/Controllo ripetitivo/Controllo ripetitivo/Regolatore ripetitivo/Ripetitivo Modulazione AM/notch_f_am/notch_demodulazione_5_7 ==
  In1 : Inport
  Discrete Transfer Fcn1 : DiscreteTransferFcn  Numerator=cell2mat(Notch_z_AM1.num)  Denominator=cell2mat(Notch_z_AM1.den)
  Out1 : Outport
  wires:
  Discrete Transfer Fcn1/1 -> Out1/1
  In1/1 -> Discrete Transfer Fcn1/1

== system Filter_attivo/Controllo tensione/Controllo ripetitivo/Controllo ripetitivo/Regolatore ripetitivo/vecchi controlli/ Ripetitivo buffer intero/Scope ==
  1 : Inport
  2 : Inport  Port=2
  3 : Inport  Port=3
  " 1 " : DataTypeConversion  SaturateOnIntegerOverflow=on  RndMeth=Zero
  " 2 " : DataTypeConversion  SaturateOnIntegerOverflow=on  RndMeth=Zero
  " 3 " : DataTypeConversion  SaturateOnIntegerOverflow=on  RndMeth=Zero
  " InputMux " : Mux  Inputs=3
  " S-Function " : S-Function  FunctionName=plecs  SFunctionDeploymentMode=off  EnableBusSupport=off
  wires:
  " InputMux "/1 -> " S-Function "/1
  1/1 -> " 1 "/1
  " 1 "/1 -> " InputMux "/1
  2/1 -> " 2 "/1
  " 2 "/1 -> " InputMux "/2
  3/1 -> " 3 "/1
  " 3 "/1 -> " InputMux "/3

== system Filter_attivo/Controllo tensione/Controllo ripetitivo/Controllo ripetitivo/Regolatore ripetitivo/vecchi controlli/ Ripetitivo buffer intero/k_serie step ==
  In1 : Inport
  Constant : Constant  Value=Tc
  Constant1 : Constant  Value=k_serie_partenza
  Constant2 : Constant  Value=passo_t
  Constant3 : Constant  Value=passo_y
  MATLAB Function : MATLAB Function  TreatAsAtomicUnit=on
  Product : Product
  Out1 : Outport
  wires:
  Constant/1 -> MATLAB Function/1(Tc)
  Constant2/1 -> MATLAB Function/3(step_t)
  Constant1/1 -> MATLAB Function/2(k_partenza)
  Constant3/1 -> MATLAB Function/4(step_y)
  In1/1 -> Product/1
  MATLAB Function/1(k) -> Product/2
  Product/1 -> Out1/1

== system Filter_attivo/Controllo tensione/Controllo ripetitivo/Controllo ripetitivo/Regolatore ripetitivo/vecchi controlli/ Ripetitivo buffer intero1.5 di ritardo/Scope ==
  1 : Inport
  2 : Inport  Port=2
  3 : Inport  Port=3
  " 1 " : DataTypeConversion  SaturateOnIntegerOverflow=on  RndMeth=Zero
  " 2 " : DataTypeConversion  SaturateOnIntegerOverflow=on  RndMeth=Zero
  " 3 " : DataTypeConversion  SaturateOnIntegerOverflow=on  RndMeth=Zero
  " InputMux " : Mux  Inputs=3
  " S-Function " : S-Function  FunctionName=plecs  SFunctionDeploymentMode=off  EnableBusSupport=off
  wires:
  " 3 "/1 -> " InputMux "/3
  3/1 -> " 3 "/1
  " 2 "/1 -> " InputMux "/2
  2/1 -> " 2 "/1
  " 1 "/1 -> " InputMux "/1
  1/1 -> " 1 "/1
  " InputMux "/1 -> " S-Function "/1

== system Filter_attivo/Controllo tensione/Controllo ripetitivo/Controllo ripetitivo/Regolatore ripetitivo/vecchi controlli/ Ripetitivo buffer intero1.5 di ritardo/k_serie step ==
  In1 : Inport
  Constant : Constant  Value=Tc
  Constant1 : Constant  Value=k_serie_partenza
  Constant2 : Constant  Value=passo_t
  Constant3 : Constant  Value=passo_y
  MATLAB Function : MATLAB Function  TreatAsAtomicUnit=on
  Product : Product
  Out1 : Outport
  wires:
  Product/1 -> Out1/1
  MATLAB Function/1(k) -> Product/2
  In1/1 -> Product/1
  Constant3/1 -> MATLAB Function/4(step_y)
  Constant1/1 -> MATLAB Function/2(k_partenza)
  Constant2/1 -> MATLAB Function/3(step_t)
  Constant/1 -> MATLAB Function/1(Tc)

== system Filter_attivo/Controllo tensione/Controllo ripetitivo/Controllo ripetitivo/Regolatore ripetitivo/vecchi controlli/ Ripetitivo stazionario/Scope ==
  1 : Inport
  2 : Inport  Port=2
  3 : Inport  Port=3
  " 1 " : DataTypeConversion  SaturateOnIntegerOverflow=on  RndMeth=Zero
  " 2 " : DataTypeConversion  SaturateOnIntegerOverflow=on  RndMeth=Zero
  " 3 " : DataTypeConversion  SaturateOnIntegerOverflow=on  RndMeth=Zero
  " InputMux " : Mux  Inputs=3
  " S-Function " : S-Function  FunctionName=plecs  SFunctionDeploymentMode=off  EnableBusSupport=off
  wires:
  " 3 "/1 -> " InputMux "/3
  3/1 -> " 3 "/1
  " 2 "/1 -> " InputMux "/2
  2/1 -> " 2 "/1
  " 1 "/1 -> " InputMux "/1
  1/1 -> " 1 "/1
  " InputMux "/1 -> " S-Function "/1

== system Filter_attivo/Controllo tensione/Controllo ripetitivo/Controllo ripetitivo/Regolatore ripetitivo/vecchi controlli/ buffer intero mattavelli buchi amplificati/Scope ==
  1 : Inport
  " InputMux " : Subsystem
      mask Display: disp('Mux')
  " S-Function " : S-Function  FunctionName=plecs  SFunctionDeploymentMode=off  EnableBusSupport=off
  wires:
  " InputMux "/1(Out) -> " S-Function "/1
  1/1 -> " InputMux "/1(In1)

== system Filter_attivo/Controllo tensione/Controllo ripetitivo/Controllo ripetitivo/Regolatore ripetitivo/vecchi controlli/ buffer intero mattavelli buchi amplificati/k_serie step ==
  In1 : Inport
  Constant : Constant  Value=Tc
  Constant1 : Constant  Value=k_serie_partenza
  Constant2 : Constant  Value=passo_t
  Constant3 : Constant  Value=passo_y
  MATLAB Function : MATLAB Function  TreatAsAtomicUnit=on
  Product : Product
  Out1 : Outport
  wires:
  Constant/1 -> MATLAB Function/1(Tc)
  Constant2/1 -> MATLAB Function/3(step_t)
  Constant1/1 -> MATLAB Function/2(k_partenza)
  Constant3/1 -> MATLAB Function/4(step_y)
  In1/1 -> Product/1
  MATLAB Function/1(k) -> Product/2
  Product/1 -> Out1/1

== system Filter_attivo/Controllo tensione/Controllo ripetitivo/Controllo ripetitivo/Regolatore ripetitivo/vecchi controlli/Ripetitivo Modulazione AM1/Banco di ripetitivi ==
  In1 : Inport
  Subsystem : Subsystem  mask{abilitatore5=1, abilitatore7=1, abilitatore11=1, abilitatore13=1, abilitatore17=1, abilitatore19=1}
      mask prompts: abilitatore5 "5^a armonica"; abilitatore7 "7^a armonica"; abilitatore11 "11^ armonica"; abilitatore13 "13^ armonica"; abilitatore17 "17^ armonica"; abilitatore19 "19^ armonica"
  rep_comp 1 : Subsystem  mask{ro=5+round(f_am/50), g_interno=10, rit=2}
      mask prompts: ro "Harmonic order"; g_interno "guadagno serie"; rit "ritardo inverter"
  rep_comp 2 : Subsystem  mask{ro=7+round(f_am/50), g_interno=5, rit=2}
      mask prompts: ro "Harmonic order"; g_interno "guadagno serie"; rit "ritardo inverter"
  rep_comp 3 : Subsystem  mask{ro=11+round(f_am/50), g_interno=1, rit=2}
      mask prompts: ro "Harmonic order"; g_interno "guadagno serie"; rit "ritardo inverter"
  rep_comp 4 : Subsystem  mask{ro=13+round(f_am/50), g_interno=1, rit=2}
      mask prompts: ro "Harmonic order"; g_interno "guadagno serie"; rit "ritardo inverter"
  rep_comp 5 : Subsystem  mask{ro=17+round(f_am/50), g_interno=0.5, rit=2}
      mask prompts: ro "Harmonic order"; g_interno "guadagno serie"; rit "ritardo inverter"
  rep_comp 6 : Subsystem  mask{ro=19+round(f_am/50), g_interno=0.5, rit=2}
      mask prompts: ro "Harmonic order"; g_interno "guadagno serie"; rit "ritardo inverter"
  Out1 : Outport
  wires:
  rep_comp 6/1(Out1) -> Subsystem/6(In6)
  rep_comp 5/1(Out1) -> Subsystem/5(In5)
  rep_comp 4/1(Out1) -> Subsystem/4(In4)
  rep_comp 3/1(Out1) -> Subsystem/3(In3)
  rep_comp 2/1(Out1) -> Subsystem/2(In2)
  rep_comp 1/1(Out1) -> Subsystem/1(In1)
  Subsystem/1(Out1) -> Out1/1
  In1/1 -> rep_comp 1/1(In1), rep_comp 2/1(In1), rep_comp 5/1(In1), rep_comp 6/1(In1), rep_comp 4/1(In1), rep_comp 3/1(In1)

== system Filter_attivo/Controllo tensione/Controllo ripetitivo/Controllo ripetitivo/Regolatore ripetitivo/vecchi controlli/Ripetitivo Modulazione AM1/Banco notch 5_7_AM ==
  In2 : Inport
  Demux1 : Demux  Outputs=2
  Mux1 : Mux  Inputs=2
  notch_demodulazione_5_1 : Subsystem
  notch_demodulazione_5_7 : Subsystem
  Out1 : Outport
  wires:
  Demux1/2 -> notch_demodulazione_5_1/1(In1)
  In2/1 -> Demux1/1
  notch_demodulazione_5_1/1(Out1) -> Mux1/2
  notch_demodulazione_5_7/1(Out1) -> Mux1/1
  Demux1/1 -> notch_demodulazione_5_7/1(In1)
  Mux1/1 -> Out1/1

== system Filter_attivo/Controllo tensione/Controllo ripetitivo/Controllo ripetitivo/Regolatore ripetitivo/vecchi controlli/Ripetitivo Modulazione AM1/Integratore discreto con reset a 2*pi ==
  omega : Inport
  Add : Sum
  Compare To Zero : simulink/Logic and Bit Operations/Compare To Zero  relop=>  OutDataTypeStr=uint8  ZeroCross=off
  Constant : Constant  Value=2*pi
  Constant1 : Constant  Value=-2*pi
  Constant2 : Constant  Value=-2*pi
  Constant3 : Constant  Value=2*pi
  Discrete-Time Integrator : DiscreteIntegrator  ExternalReset=rising  InitialConditionSource=external  SampleTime=-1  ShowStatePort=on  ICPrevOutput=DiscIntNeverNeededParam  ICPrevScaledInput=DiscIntNeverNeededParam
  Logical Operator2 : Logic  Operator=OR  AllPortsSameDT=off  OutDataTypeStr=boolean
  Relational Operator : RelationalOperator  Operator=<=  OutDataTypeStr=boolean  RndMeth=Nearest
  Relational Operator1 : RelationalOperator  Operator=<=  OutDataTypeStr=boolean  RndMeth=Nearest
  Switch : Switch  Threshold=0.5
  teta : Outport
  wires:
  Add/1 -> Discrete-Time Integrator/3
  Compare To Zero/1 -> Switch/2
  Switch/1 -> Add/2
  Constant3/1 -> Switch/3
  Constant2/1 -> Switch/1
  Discrete-Time Integrator/1 -> teta/1
  omega/1 -> Discrete-Time Integrator/1
  Constant1/1 -> Relational Operator1/2
  Constant/1 -> Relational Operator/1
  Discrete-Time Integrator/State -> Relational Operator/2, Relational Operator1/1, Compare To Zero/1, Add/1
  Relational Operator1/1 -> Logical Operator2/2
  Relational Operator/1 -> Logical Operator2/1
  Logical Operator2/1 -> Discrete-Time Integrator/2

== system Filter_attivo/Controllo tensione/Controllo ripetitivo/Controllo ripetitivo/Regolatore ripetitivo/vecchi controlli/Ripetitivo Modulazione AM1/Scope ==
  1 : Inport
  2 : Inport  Port=2
  3 : Inport  Port=3
  " 1 " : DataTypeConversion  SaturateOnIntegerOverflow=on  RndMeth=Zero
  " 2 " : DataTypeConversion  SaturateOnIntegerOverflow=on  RndMeth=Zero
  " 3 " : DataTypeConversion  SaturateOnIntegerOverflow=on  RndMeth=Zero
  " InputMux " : Mux  Inputs=3
  " S-Function " : S-Function  FunctionName=plecs  SFunctionDeploymentMode=off  EnableBusSupport=off
  wires:
  " 3 "/1 -> " InputMux "/3
  3/1 -> " 3 "/1
  " 2 "/1 -> " InputMux "/2
  2/1 -> " 2 "/1
  " 1 "/1 -> " InputMux "/1
  1/1 -> " 1 "/1
  " InputMux "/1 -> " S-Function "/1

== system Filter_attivo/Controllo tensione/Controllo ripetitivo/Controllo ripetitivo/Regolatore ripetitivo/vecchi controlli/Ripetitivo Modulazione AM1/Scope1 ==
  1 : Inport
  " InputMux " : Subsystem
      mask Display: disp('Mux')
  " S-Function " : S-Function  FunctionName=plecs  SFunctionDeploymentMode=off  EnableBusSupport=off
  wires:
  " InputMux "/1(Out) -> " S-Function "/1
  1/1 -> " InputMux "/1(In1)

== system Filter_attivo/Controllo tensione/Controllo ripetitivo/Controllo ripetitivo con downsampling/Regolatore ripetitivo/ buffer metà mattavelli/Scope/ InputMux  ==
  In1 : Inport
  Convert1 : DataTypeConversion  SaturateOnIntegerOverflow=on  RndMeth=Zero
  Mux : Mux  Inputs=1
  Out : Outport
  wires:
  Mux/1 -> Out/1
  In1/1 -> Convert1/1
  Convert1/1 -> Mux/1

== system Filter_attivo/Controllo tensione/Controllo PR 10 kHz/PLL_tempo_discreto/Subsystem/notch_prima_tensione/FILTRO peaking diretta_prima/Scope/ InputMux  ==
  In1 : Inport
  Convert1 : DataTypeConversion  SaturateOnIntegerOverflow=on  RndMeth=Zero
  Mux : Mux  Inputs=1
  Out : Outport
  wires:
  Convert1/1 -> Mux/1
  In1/1 -> Convert1/1
  Mux/1 -> Out/1

== system Filter_attivo/Controllo tensione/Controllo ripetitivo/Controllo ripetitivo/Regolatore ripetitivo/Ripetitivo Modulazione AM/Banco di ripetitivi/rep_comp 1/Scope2 ==
  1 : Inport
  " InputMux " : Subsystem
      mask Display: disp('Mux')
  " S-Function " : S-Function  FunctionName=plecs  SFunctionDeploymentMode=off  EnableBusSupport=off
  wires:
  " InputMux "/1(Out) -> " S-Function "/1
  1/1 -> " InputMux "/1(In1)

== system Filter_attivo/Controllo tensione/Controllo ripetitivo/Controllo ripetitivo/Regolatore ripetitivo/Ripetitivo Modulazione AM/Banco di ripetitivi/rep_comp 2/Scope2 ==
  1 : Inport
  " InputMux " : Subsystem
      mask Display: disp('Mux')
  " S-Function " : S-Function  FunctionName=plecs  SFunctionDeploymentMode=off  EnableBusSupport=off
  wires:
  1/1 -> " InputMux "/1(In1)
  " InputMux "/1(Out) -> " S-Function "/1

== system Filter_attivo/Controllo tensione/Controllo ripetitivo/Controllo ripetitivo/Regolatore ripetitivo/Ripetitivo Modulazione AM/Banco di ripetitivi/rep_comp 3/Scope2 ==
  1 : Inport
  " InputMux " : Subsystem
      mask Display: disp('Mux')
  " S-Function " : S-Function  FunctionName=plecs  SFunctionDeploymentMode=off  EnableBusSupport=off
  wires:
  " InputMux "/1(Out) -> " S-Function "/1
  1/1 -> " InputMux "/1(In1)

== system Filter_attivo/Controllo tensione/Controllo ripetitivo/Controllo ripetitivo/Regolatore ripetitivo/Ripetitivo Modulazione AM/Banco di ripetitivi/rep_comp 4/Scope2 ==
  1 : Inport
  " InputMux " : Subsystem
      mask Display: disp('Mux')
  " S-Function " : S-Function  FunctionName=plecs  SFunctionDeploymentMode=off  EnableBusSupport=off
  wires:
  1/1 -> " InputMux "/1(In1)
  " InputMux "/1(Out) -> " S-Function "/1

== system Filter_attivo/Controllo tensione/Controllo ripetitivo/Controllo ripetitivo/Regolatore ripetitivo/Ripetitivo Modulazione AM/Banco di ripetitivi/rep_comp 5/Scope2 ==
  1 : Inport
  " InputMux " : Subsystem
      mask Display: disp('Mux')
  " S-Function " : S-Function  FunctionName=plecs  SFunctionDeploymentMode=off  EnableBusSupport=off
  wires:
  " InputMux "/1(Out) -> " S-Function "/1
  1/1 -> " InputMux "/1(In1)

== system Filter_attivo/Controllo tensione/Controllo ripetitivo/Controllo ripetitivo/Regolatore ripetitivo/Ripetitivo Modulazione AM/Banco di ripetitivi/rep_comp 6/Scope2 ==
  1 : Inport
  " InputMux " : Subsystem
      mask Display: disp('Mux')
  " S-Function " : S-Function  FunctionName=plecs  SFunctionDeploymentMode=off  EnableBusSupport=off
  wires:
  1/1 -> " InputMux "/1(In1)
  " InputMux "/1(Out) -> " S-Function "/1

== system Filter_attivo/Controllo tensione/Controllo ripetitivo/Controllo ripetitivo/Regolatore ripetitivo/vecchi controlli/ buffer intero mattavelli buchi amplificati/Scope/ InputMux  ==
  In1 : Inport
  Convert1 : DataTypeConversion  SaturateOnIntegerOverflow=on  RndMeth=Zero
  Mux : Mux  Inputs=1
  Out : Outport
  wires:
  Mux/1 -> Out/1
  In1/1 -> Convert1/1
  Convert1/1 -> Mux/1

== system Filter_attivo/Controllo tensione/Controllo ripetitivo/Controllo ripetitivo/Regolatore ripetitivo/vecchi controlli/Ripetitivo Modulazione AM1/Banco di ripetitivi/Subsystem ==
  In1 : Inport
  In2 : Inport  Port=2
  In3 : Inport  Port=3
  In4 : Inport  Port=4
  In5 : Inport  Port=5
  In6 : Inport  Port=6
  Gain : Gain  Gain=abilitatore5
  Gain1 : Gain  Gain=abilitatore7
  Gain2 : Gain  Gain=abilitatore13
  Gain3 : Gain  Gain=abilitatore11
  Gain4 : Gain  Gain=abilitatore17
  Gain5 : Gain  Gain=abilitatore19
  Sum : Sum  Inputs=++++++
  Out1 : Outport
  wires:
  Gain5/1 -> Sum/6
  Gain4/1 -> Sum/5
  Gain2/1 -> Sum/4
  Gain3/1 -> Sum/3
  Gain1/1 -> Sum/2
  Gain/1 -> Sum/1
  Sum/1 -> Out1/1
  In6/1 -> Gain5/1
  In4/1 -> Gain2/1
  In2/1 -> Gain1/1
  In1/1 -> Gain/1
  In3/1 -> Gain3/1
  In5/1 -> Gain4/1

== system Filter_attivo/Controllo tensione/Controllo ripetitivo/Controllo ripetitivo/Regolatore ripetitivo/vecchi controlli/Ripetitivo Modulazione AM1/Banco di ripetitivi/rep_comp 1 ==
  In1 : Inport
  Add1 : Sum  Inputs=-+
  Delay1 : Delay
  Delay3 : Delay  DelayLength=fix(1/(Tc*f*1*ro)-1-rit)
  Discrete FIR Filter : DiscreteFir  Coefficients=[h(1,ro) h(2,ro) h(3,ro) h(4,ro)]
  Gain : Gain  Gain=0.98
  Gain1 : Gain  Gain=g_interno
  Scope2 : Subsystem  LoadFcn=plecs('sl', 300);  InitFcn=plecs('sl', 314);  StartFcn=plecs('sl', 308);  StopFcn=plecs('sl', 309);  mask{Settings=<binary blob, 216 chars, not shown>}
      mask init:
      | plecs('sl', 315);
      settings: CopyFcn=plecs('sl', 303);  DeleteFcn=plecs('sl', 305);  UndoDeleteFcn=plecs('sl', 306);  PreSaveFcn=plecs('sl', 311);  NameChangeFcn=plecs('sl', 310);  DestroyFcn=plecs('sl', 307);  OpenFcn=plecs('sl', 302);  ErrorFcn=plerrorfcn
      mask Display: plot([0.1 0.9 0.9 0.1 0.1], [0.9 0.9 0.5 0.5 0.9])
  Out1 : Outport
  wires:
  Gain1/1 -> Out1/1, Scope2/1(1)
  Discrete FIR Filter/1 -> Gain/1, Gain1/1
  Gain/1 -> Delay1/1
  Delay1/1 -> Add1/2
  Add1/1 -> Delay3/1
  In1/1 -> Add1/1
  Delay3/1 -> Discrete FIR Filter/1

== system Filter_attivo/Controllo tensione/Controllo ripetitivo/Controllo ripetitivo/Regolatore ripetitivo/vecchi controlli/Ripetitivo Modulazione AM1/Banco di ripetitivi/rep_comp 2 ==
  In1 : Inport
  Add1 : Sum  Inputs=-+
  Delay1 : Delay
  Delay3 : Delay  DelayLength=fix(1/(Tc*f*1*ro)-1-rit)
  Discrete FIR Filter : DiscreteFir  Coefficients=[h(1,ro) h(2,ro) h(3,ro) h(4,ro)]
  Gain : Gain  Gain=0.98
  Gain1 : Gain  Gain=g_interno
  Scope2 : Subsystem  LoadFcn=plecs('sl', 300);  InitFcn=plecs('sl', 314);  StartFcn=plecs('sl', 308);  StopFcn=plecs('sl', 309);  mask{Settings=<binary blob, 216 chars, not shown>}
      mask init:
      | plecs('sl', 315);
      settings: CopyFcn=plecs('sl', 303);  DeleteFcn=plecs('sl', 305);  UndoDeleteFcn=plecs('sl', 306);  PreSaveFcn=plecs('sl', 311);  NameChangeFcn=plecs('sl', 310);  DestroyFcn=plecs('sl', 307);  OpenFcn=plecs('sl', 302);  ErrorFcn=plerrorfcn
      mask Display: plot([0.1 0.9 0.9 0.1 0.1], [0.9 0.9 0.5 0.5 0.9])
  Out1 : Outport
  wires:
  Delay3/1 -> Discrete FIR Filter/1
  In1/1 -> Add1/1
  Add1/1 -> Delay3/1
  Delay1/1 -> Add1/2
  Gain/1 -> Delay1/1
  Discrete FIR Filter/1 -> Gain1/1, Gain/1
  Gain1/1 -> Scope2/1(1), Out1/1

== system Filter_attivo/Controllo tensione/Controllo ripetitivo/Controllo ripetitivo/Regolatore ripetitivo/vecchi controlli/Ripetitivo Modulazione AM1/Banco di ripetitivi/rep_comp 3 ==
  In1 : Inport
  Add1 : Sum  Inputs=-+
  Delay1 : Delay
  Delay3 : Delay  DelayLength=fix(1/(Tc*f*1*ro)-1-rit)
  Discrete FIR Filter : DiscreteFir  Coefficients=[h(1,ro) h(2,ro) h(3,ro) h(4,ro)]
  Gain : Gain  Gain=0.98
  Gain1 : Gain  Gain=g_interno
  Scope2 : Subsystem  LoadFcn=plecs('sl', 300);  InitFcn=plecs('sl', 314);  StartFcn=plecs('sl', 308);  StopFcn=plecs('sl', 309);  mask{Settings=<binary blob, 216 chars, not shown>}
      mask init:
      | plecs('sl', 315);
      settings: CopyFcn=plecs('sl', 303);  DeleteFcn=plecs('sl', 305);  UndoDeleteFcn=plecs('sl', 306);  PreSaveFcn=plecs('sl', 311);  NameChangeFcn=plecs('sl', 310);  DestroyFcn=plecs('sl', 307);  OpenFcn=plecs('sl', 302);  ErrorFcn=plerrorfcn
      mask Display: plot([0.1 0.9 0.9 0.1 0.1], [0.9 0.9 0.5 0.5 0.9])
  Out1 : Outport
  wires:
  Gain1/1 -> Out1/1, Scope2/1(1)
  Discrete FIR Filter/1 -> Gain/1, Gain1/1
  Gain/1 -> Delay1/1
  Delay1/1 -> Add1/2
  Add1/1 -> Delay3/1
  In1/1 -> Add1/1
  Delay3/1 -> Discrete FIR Filter/1

== system Filter_attivo/Controllo tensione/Controllo ripetitivo/Controllo ripetitivo/Regolatore ripetitivo/vecchi controlli/Ripetitivo Modulazione AM1/Banco di ripetitivi/rep_comp 4 ==
  In1 : Inport
  Add1 : Sum  Inputs=-+
  Delay1 : Delay
  Delay3 : Delay  DelayLength=fix(1/(Tc*f*1*ro)-1-rit)
  Discrete FIR Filter : DiscreteFir  Coefficients=[h(1,ro) h(2,ro) h(3,ro) h(4,ro)]
  Gain : Gain  Gain=0.98
  Gain1 : Gain  Gain=g_interno
  Scope2 : Subsystem  LoadFcn=plecs('sl', 300);  InitFcn=plecs('sl', 314);  StartFcn=plecs('sl', 308);  StopFcn=plecs('sl', 309);  mask{Settings=<binary blob, 216 chars, not shown>}
      mask init:
      | plecs('sl', 315);
      settings: CopyFcn=plecs('sl', 303);  DeleteFcn=plecs('sl', 305);  UndoDeleteFcn=plecs('sl', 306);  PreSaveFcn=plecs('sl', 311);  NameChangeFcn=plecs('sl', 310);  DestroyFcn=plecs('sl', 307);  OpenFcn=plecs('sl', 302);  ErrorFcn=plerrorfcn
      mask Display: plot([0.1 0.9 0.9 0.1 0.1], [0.9 0.9 0.5 0.5 0.9])
  Out1 : Outport
  wires:
  Delay3/1 -> Discrete FIR Filter/1
  In1/1 -> Add1/1
  Add1/1 -> Delay3/1
  Delay1/1 -> Add1/2
  Gain/1 -> Delay1/1
  Discrete FIR Filter/1 -> Gain1/1, Gain/1
  Gain1/1 -> Scope2/1(1), Out1/1
